simulink model "e03_MtrCtrl_MtrCtrl"  (R2024a)
settings: Solver=FixedStepDiscrete  StartTime=0.0  StopTime=1  FixedStep=mSim.dTime  MaxStep=Define.sModelSampleTime  RelTol=7.1420e-05
undefined symbols (not defined in the file): CnstCnst, CnstMde, CnstNr, E03CCTRL, E03INIT, E03LIM, E03MCMV, sTempGain
libraries: Lib_LPF x2
(part 3 of 3)

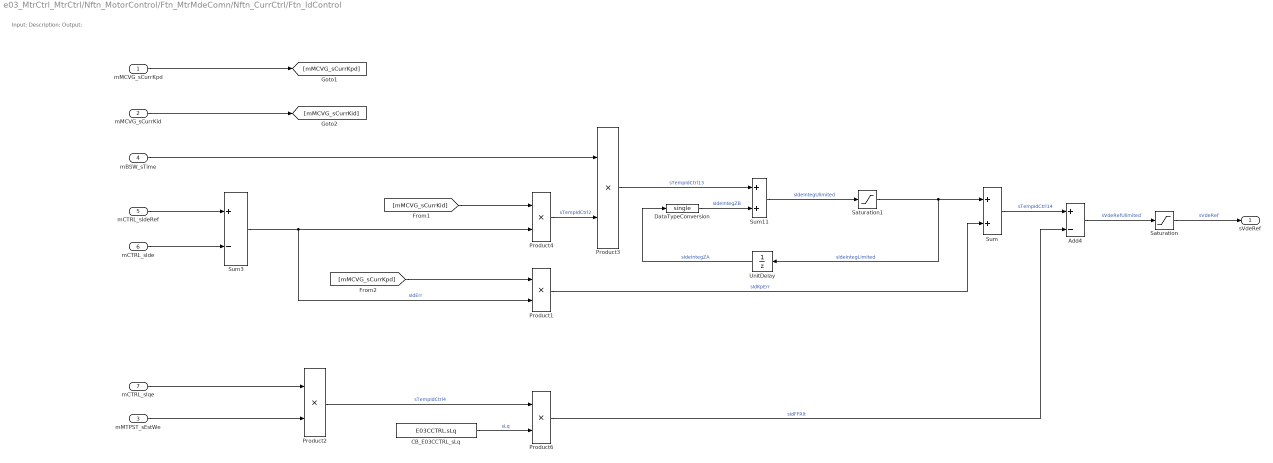
== system e03_MtrCtrl_MtrCtrl/Nftn_MotorControl/Ftn_MtrMdeComn/Nftn_CurrCtrl/Ftn_IdControl ==
  note: Input:
      | Description:
      | Output:
  mMCVG_sCurrKpd : Inport  Description=■ 설명: Current Gain Kp Gain  OutMin=0  OutMax=100
      settings: AttributesFormatString=%<Description>
  mMCVG_sCurrKid : Inport  Description=■ 설명: Current Gain Ki Gain  Port=2  OutMin=0  OutMax=100
      settings: AttributesFormatString=%<Description>
  mMTPST_sEstWe : Inport  Description=■ 설명: 전기 각속도 (We = Wm * Poles)  Port=3  OutMin=0  OutMax=5026.55
      settings: AttributesFormatString=%<Description>
  mBSW_sTime : Inport  Description=■ 설명: 주기, sTime (1/14kH)  Port=4  OutMin=0  OutMax=0.0000714286
      settings: AttributesFormatString=%<Description>
  mCTRL_sIdeRef : Inport  Description=■ 설명: d축 전류 지령  Port=5  OutMin=-49.498  OutMax=49.498
      settings: AttributesFormatString=%<Description>
  mCTRL_sIde : Inport  Description=■ 설명: d축 전류  Port=6  OutMin=-398.3  OutMax=398.3
      settings: AttributesFormatString=%<Description>
  mCTRL_sIqe : Inport  Description=■ 설명: q축 전류  Port=7  OutMin=-398.3  OutMax=398.3
      settings: AttributesFormatString=%<Description>
  Add4 : Sum  Inputs=+-
  CB_E03CCTRL_sLq : Constant  Value=E03CCTRL.sLq
  DataTypeConversion : DataTypeConversion  OutDataTypeStr=single  SaturateOnIntegerOverflow=off  RndMeth=Floor
  Product{1..4,6} (5 alike) : Product
  Saturation : Saturate  UpperLimit=E03LIM.sVrefLim  LowerLimit=E03LIM.sNegVrefLim
      settings: AttributesFormatString=|
      | %<LowerLimit>
      | %<UpperLimit>
  Saturation1 : Saturate  UpperLimit=E03LIM.sVrefLim  LowerLimit=E03LIM.sNegVrefLim
      settings: AttributesFormatString=|
      | %<LowerLimit>
      | %<UpperLimit>
  Sum : Sum
  Sum11 : Sum
  Sum3 : Sum  Inputs=+-
  UnitDelay : UnitDelay  InitialCondition=E03INIT.sIdeCtrlIntegZ  SampleTime=-1  StateName=sIdeIntegZ  HasFrameUpgradeWarning=on
      settings: AttributesFormatString=%<InitialCondition>
  sVdeRef : Outport  Description=■ 설명: d축 전압 지령  OutMin=-1000  OutMax=1000  VectorParamsAs1DForOutWhenUnconnected=off
      settings: AttributesFormatString=%<Description>
  wires:
  Saturation1/1 -> Sum/1, UnitDelay/1  "sIdeIntegLimited"
  Add4/1 -> Saturation/1  "sVdeRefUlimited"
  Product4/1 -> Product3/2  "sTempIdCtrl2"
  Sum3/1 -> Product1/2, Product4/2  "sIdErr"
  Product2/1 -> Product6/1  "sTempIdCtrl4"
  Product1/1 -> Sum/2  "sIdKpErr"
  Product3/1 -> Sum11/1  "sTempIdCtrl13"
  UnitDelay/1 -> DataTypeConversion/1  "sIdeIntegZA"
  mBSW_sTime/1 -> Product3/1
  CB_E03CCTRL_sLq/1 -> Product6/2  "sLq"
  Sum/1 -> Add4/1  "sTempIdCtrl14"
  [mMCVG_sCurrKpd] -> Product1/1
  [mMCVG_sCurrKid] -> Product4/1
  DataTypeConversion/1 -> Sum11/2  "sIdeIntegZB"
  Saturation/1 -> sVdeRef/1  "sVdeRef"
  mMCVG_sCurrKpd/1 -> [mMCVG_sCurrKpd]
  mMCVG_sCurrKid/1 -> [mMCVG_sCurrKid]
  mCTRL_sIdeRef/1 -> Sum3/1
  mCTRL_sIde/1 -> Sum3/2
  mCTRL_sIqe/1 -> Product2/1
  mMTPST_sEstWe/1 -> Product2/2
  Sum11/1 -> Saturation1/1  "sIdeIntegUlimited"
  Product6/1 -> Add4/2  "sIdFFRlt"

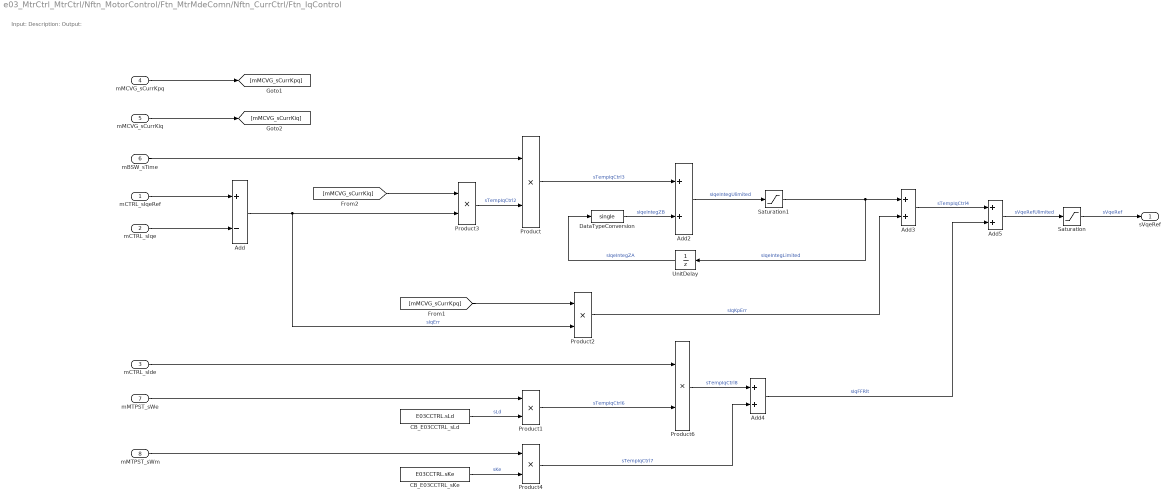
== system e03_MtrCtrl_MtrCtrl/Nftn_MotorControl/Ftn_MtrMdeComn/Nftn_CurrCtrl/Ftn_IqControl ==
  note: Input:
      | Description:
      | Output:
  mCTRL_sIqeRef : Inport  Description=■ 설명: q축 전류 지령  OutMin=-49.498  OutMax=49.498
      settings: AttributesFormatString=%<Description>
  mCTRL_sIqe : Inport  Description=■ 설명: q축 전류  Port=2  OutMin=-398.3  OutMax=398.3
      settings: AttributesFormatString=%<Description>
  mCTRL_sIde : Inport  Description=■ Ide 전류  Port=3  OutMin=-398.3  OutMax=398.3
      settings: AttributesFormatString=%<Description>
  mMCVG_sCurrKpq : Inport  Description=■ 설명: Current Gain Kp Gain  Port=4  OutMin=0  OutMax=100
      settings: AttributesFormatString=%<Description>
  mMCVG_sCurrKiq : Inport  Description=■ 설명: Current Gain Ki Gain  Port=5  OutMin=0  OutMax=100
      settings: AttributesFormatString=%<Description>
  mBSW_sTime : Inport  Description=■ 설명: 주기, sTime (1/14kH)  Port=6  OutMin=0  OutMax=0.0000714286
      settings: AttributesFormatString=%<Description>
  mMTPST_sWe : Inport  Description=■ 설명: 전기 각속도 (We = Wm * Poles)  Port=7  OutMin=0  OutMax=5026.55
      settings: AttributesFormatString=%<Description>
  mMTPST_sWm : Inport  Description=■ 설명: 기계 각속도 (Wm = 12000 * 2pi/60)  Port=8  OutMin=0  OutMax=1256.63706
      settings: AttributesFormatString=%<Description>
  Add : Sum  Inputs=+-
  Add{2..5} (4 alike) : Sum
  CB_E03CCTRL_sKe : Constant  Value=E03CCTRL.sKe
  CB_E03CCTRL_sLd : Constant  Value=E03CCTRL.sLd
  DataTypeConversion : DataTypeConversion  OutDataTypeStr=single  SaturateOnIntegerOverflow=off  RndMeth=Floor
  Product{,1..4,6} (6 alike) : Product
  Saturation : Saturate  UpperLimit=E03LIM.sVrefLim  LowerLimit=E03LIM.sNegVrefLim
      settings: AttributesFormatString=|
      | %<LowerLimit>
      | %<UpperLimit>
  Saturation1 : Saturate  UpperLimit=E03LIM.sVrefLim  LowerLimit=E03LIM.sNegVrefLim
      settings: AttributesFormatString=|
      | %<LowerLimit>
      | %<UpperLimit>
  UnitDelay : UnitDelay  InitialCondition=E03INIT.sIqeCtrlIntegZ  SampleTime=-1  StateName=sIqeIntegZ  HasFrameUpgradeWarning=on
      settings: AttributesFormatString=%<InitialCondition>
  sVqeRef : Outport  Description=■ 설명: q축 전압 지령  OutMin=-1000  OutMax=1000  VectorParamsAs1DForOutWhenUnconnected=off
      settings: AttributesFormatString=%<Description>
  wires:
  Add3/1 -> Add5/1  "sTempIqCtrl4"
  Add/1 -> Product2/2, Product3/2  "sIqErr"
  Add5/1 -> Saturation/1  "sVqeRefUlimited"
  Product2/1 -> Add3/2  "sIqKpErr"
  Add4/1 -> Add5/2  "sIqFFRlt"
  Product6/1 -> Add4/1  "sTempIqCtrl8"
  Saturation1/1 -> UnitDelay/1, Add3/1  "sIqeIntegLimited"
  Product/1 -> Add2/1  "sTempIqCtrl3"
  mBSW_sTime/1 -> Product/1
  Product3/1 -> Product/2  "sTempIqCtrl2"
  [mMCVG_sCurrKiq] -> Product3/1
  Product4/1 -> Add4/2  "sTempIqCtrl7"
  CB_E03CCTRL_sLd/1 -> Product1/2  "sLd"
  CB_E03CCTRL_sKe/1 -> Product4/2  "sKe"
  Product1/1 -> Product6/2  "sTempIqCtrl6"
  [mMCVG_sCurrKpq] -> Product2/1
  UnitDelay/1 -> DataTypeConversion/1  "sIqeIntegZA"
  DataTypeConversion/1 -> Add2/2  "sIqeIntegZB"
  Saturation/1 -> sVqeRef/1  "sVqeRef"
  mMCVG_sCurrKpq/1 -> [mMCVG_sCurrKpq]
  mMCVG_sCurrKiq/1 -> [mMCVG_sCurrKiq]
  mMTPST_sWe/1 -> Product1/1
  mMTPST_sWm/1 -> Product4/1
  mCTRL_sIqeRef/1 -> Add/1
  mCTRL_sIqe/1 -> Add/2
  mCTRL_sIde/1 -> Product6/1
  Add2/1 -> Saturation1/1  "sIqeIntegUlimited"

== system e03_MtrCtrl_MtrCtrl/Nftn_MotorControl/Ftn_MtrMdeComn/Nftn_CurrCtrl/Nftn_GenMuxVdqeRef ==
  note: Input:
      | Description:
      | Output:
  sVdeRef : Inport
  sTheta : Inport  Port=2
  sVqeRef : Inport  Port=3
  Mux : Mux  Inputs=3
  sVdqeRef : Outport
  wires:
  Mux/1 -> sVdqeRef/1  "sVdqeRef"
  sTheta/1 -> Mux/3
  sVqeRef/1 -> Mux/2
  sVdeRef/1 -> Mux/1

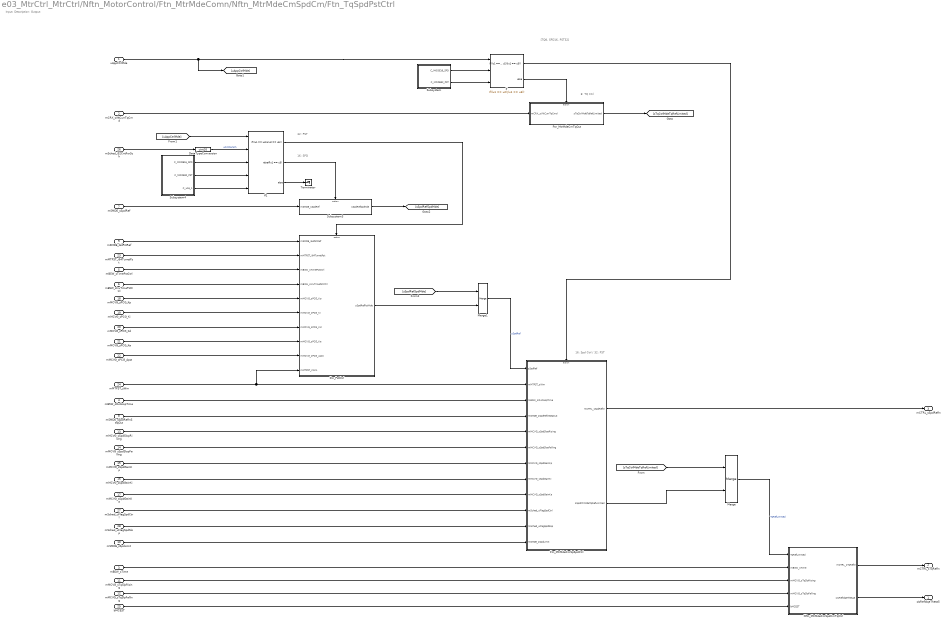
== system e03_MtrCtrl_MtrCtrl/Nftn_MotorControl/Ftn_MtrMdeComn/Nftn_MtrMdeCmSpdCm/Ftn_TqSpdPstCtrl ==
  note: 8: TQ Ctrl
  note: Input:
      | Description:
      | Output:
  note: 16: Spd Ctrl / 32: PST
  note: [TQ8, SPD16, PST32]
  note: 16: SPD
  note: 32: PST
  uAppCtrlMde : Inport  Description=■ 설명: 모터 구동 제어 모드  OutMin=0  OutMax=32
      settings: AttributesFormatString=%<Description>
  mCRX_sVltCurrTqCmd : Inport  Description=■ 설명: uVltCurrTqCmd(Voltage / Current / Torque Reference)  Port=2  OutMin=-398.3  OutMax=398.3
      settings: AttributesFormatString=%<Description>
  mBSW_sTime : Inport  Port=3
  mBSW_sOutloopTime : Inport  Description=■ 설명: sTime * 10  Port=4  OutMin=0  OutMax=0.000714286
      settings: AttributesFormatString=%<Description>
  mBSW_sTimePstCtrl : Inport  Description=■ 설명: sTime * 100  Port=5
      settings: AttributesFormatString=%<Description>
  mBSW_sInvTimePstCtrl : Inport  Description=■ 설명: mBSW_sTimePstCtrl의 역수  Port=6
      settings: AttributesFormatString=%<Description>
  mSMDE_sSpdRef : Inport  Description=■ 설명: Speed Reference  Port=7  OutMin=0  OutMax=11000
      settings: AttributesFormatString=%<Description>
  mSMDE_sSpdRefInSeqOut : Inport  Description=■ 설명: Speed Reference Slop Out  Port=8  OutMin=0  OutMax=11000
      settings: AttributesFormatString=%<Description>
  mSMDE_i64PstRef : Inport  Description='■ 설명: Position Reference  Port=9
      settings: AttributesFormatString=%<Description>
  mSMDE_sSpdLimit : Inport  Description='■ 설명: 속도 제한값  Port=10
      settings: AttributesFormatString=%<Description>
  mMCVG_sTqSlpRising : Inport  Port=11
  mMCVG_sTqSlpFalling : Inport  Port=12
  mMCVG_sSpdSlopRising : Inport  Description=■ 설명: Speed Slop Rising Gain  Port=13  OutMin=0  OutMax=3000
      settings: AttributesFormatString=%<Description>
  mMCVG_sSpdSlopFalling : Inport  Description=■ 설명: Speed Slop Falling Gain  Port=14  OutMin=0  OutMax=3000
      settings: AttributesFormatString=%<Description>
  mMCVG_sSpdGainKp : Inport  Description=■ 설명: Speed Gain Kp Gain  Port=15  OutMin=0  OutMax=10
      settings: AttributesFormatString=%<Description>
  mMCVG_sSpdGainKi : Inport  Description=■ 설명: Speed Gain Ki Gain  Port=16  OutMin=0  OutMax=10
      settings: AttributesFormatString=%<Description>
  mMCVG_sSpdGainKa : Inport  Description=■ 설명: Speed Gain Ka Gain  Port=17  OutMin=0  OutMax=100
      settings: AttributesFormatString=%<Description>
  mMCVG_sPCG_Kp : Inport  Description=■ 설명: 위치 제어 게인 Kp  Port=18
      settings: AttributesFormatString=%<Description>
  mMCVG_sPCG_Ki : Inport  Description=■ 설명: 위치 제어 게인 Ki  Port=19
      settings: AttributesFormatString=%<Description>
  mMCVG_sPCG_Kd : Inport  Description=■ 설명: 위치 제어 게인 Kd  Port=20
      settings: AttributesFormatString=%<Description>
  mMCVG_sPCG_Ka : Inport  Description=■ 설명: 위치 제어 게인 Ka  Port=21
      settings: AttributesFormatString=%<Description>
  mMCVG_sPCG_Apst : Inport  Description=■ 설명: 가속도 게인  Port=22
      settings: AttributesFormatString=%<Description>
  mMTPST_i64TurretPst : Inport  Description=■ 설명: Turret Position  Port=23
      settings: AttributesFormatString=%<Description>
  mMTPST_sWm : Inport  Description=■ 설명: 기계 각속도 (Wm = 2000 * 2pi/60)  Port=24  OutMin=0  OutMax=1256.63706
      settings: AttributesFormatString=%<Description>
  bMCEST : Inport  Port=25
  mSched_i32CntForSch : Inport  Port=26
  mSched_uFlagSpdCtrl : Inport  Description=■ 설명: Speed Control 스케쥴 카운터  Port=27  OutMin=0  OutMax=1
      settings: AttributesFormatString=%<Description>
  mSched_uFlagSpdSlop : Inport  Description=■ 설명: 속도 지령 Slop 스케쥴 카운터  Port=28  OutMin=0  OutMax=1
      settings: AttributesFormatString=%<Description>
  DataTypeConversion : DataTypeConversion  OutDataTypeStr=uint16  SaturateOnIntegerOverflow=off  RndMeth=Floor
  Ftn_MtrMdeCmSpSpdCtrl : Subsystem
      settings: RTWSystemCode=Nonreusable function  RTWFcnNameOpts=Use subsystem name
  Ftn_MtrMdeCmTqOut : Subsystem
  Ftn_PstCtrl : Subsystem
      settings: RTWSystemCode=Nonreusable function  RTWFcnNameOpts=Use subsystem name
  If : If  NumInputs=3  IfExpression=(u1 == u2)|(u1 == u3)
  If1 : If  NumInputs=5  IfExpression=(u1 == u4)&(u2 == u5)  ElseIfExpressions=u1 == u3
  Merge : Merge
  Merge1 : Merge
  Nftn_MtrMdeCmSpdCmTqCtrl : Subsystem
  Subsystem : Subsystem
  Subsystem3 : Subsystem
  Subsystem4 : Subsystem
  Terminator : Terminator
  sIsRefIdqeTheta5 : Outport  Description=|  OutMin=-398.3  OutMax=398.3
      | ■ 설명: 제어 모드 전류 출력 Mux 신호
      | -.[0] : 전압/전류/토크 지령
      | -.[1] : d축 전류
      | -.[2] : q축 전류
      | -.[3] : 추정 위치
      settings: AttributesFormatString=%<Description>
  mCTRL_sTqRefIn : Outport  Description=■ 설명: Tq Slop Reference  Port=2  OutMin=-398.3  OutMax=398.3
      settings: AttributesFormatString=%<Description>
  mCTRL_sSpdRefIn : Outport  Description=■ 설명: Speed Reference  Port=3  OutMin=0  OutMax=11000
      settings: AttributesFormatString=%<Description>
  wires:
  [sTqCtrlMdeTqRefLimited] -> Merge/1
  If/1 -> Ftn_MtrMdeCmSpSpdCtrl/Action
  uAppCtrlMde/1 -> [uAppCtrlMde], If/1
  If/2 -> Ftn_MtrMdeCmTqOut/Action
  Ftn_MtrMdeCmSpSpdCtrl/1(mCTRL_sSpdRefIn) -> mCTRL_sSpdRefIn/1
  Nftn_MtrMdeCmSpdCmTqCtrl/2(sIsRefIdqeTheta5) -> sIsRefIdqeTheta5/1
  Ftn_MtrMdeCmTqOut/1(sTqCtrlMdeTqRefLimited) -> [sTqCtrlMdeTqRefLimited]
  mBSW_sOutloopTime/1 -> Ftn_MtrMdeCmSpSpdCtrl/3(mBSW_sOutloopTime)
  mSMDE_sSpdRef/1 -> Subsystem3/1(mSMDE_sSpdRef)
  mSMDE_sSpdRefInSeqOut/1 -> Ftn_MtrMdeCmSpSpdCtrl/4(mSMDE_sSpdRefInSeqOut)
  mCRX_sVltCurrTqCmd/1 -> Ftn_MtrMdeCmTqOut/1(mCRX_sVltCurrTqCmd)
  mMCVG_sSpdSlopRising/1 -> Ftn_MtrMdeCmSpSpdCtrl/5(mMCVG_sSpdSlopRising)
  mMCVG_sSpdSlopFalling/1 -> Ftn_MtrMdeCmSpSpdCtrl/6(mMCVG_sSpdSlopFalling)
  mMCVG_sSpdGainKp/1 -> Ftn_MtrMdeCmSpSpdCtrl/7(mMCVG_sSpdGainKp)
  mMCVG_sSpdGainKi/1 -> Ftn_MtrMdeCmSpSpdCtrl/8(mMCVG_sSpdGainKi)
  mMCVG_sSpdGainKa/1 -> Ftn_MtrMdeCmSpSpdCtrl/9(mMCVG_sSpdGainKa)
  mMTPST_sWm/1 -> Ftn_PstCtrl/10(mMTPST_sWm), Ftn_MtrMdeCmSpSpdCtrl/2(mMTPST_sWm)
  mSched_uFlagSpdCtrl/1 -> Ftn_MtrMdeCmSpSpdCtrl/10(mSched_uFlagSpdCtrl)
  mSched_uFlagSpdSlop/1 -> Ftn_MtrMdeCmSpSpdCtrl/11(mSched_uFlagSpdSlop)
  bMCEST/1 -> Nftn_MtrMdeCmSpdCmTqCtrl/5(bMCEST)
  Ftn_MtrMdeCmSpSpdCtrl/2(sSpdCtrlMdeTqRefLimited) -> Merge/2
  Nftn_MtrMdeCmSpdCmTqCtrl/1(mCTRL_sTqRefIn) -> mCTRL_sTqRefIn/1
  mMCVG_sTqSlpFalling/1 -> Nftn_MtrMdeCmSpdCmTqCtrl/4(mMCVG_sTqSlpFalling)
  mMCVG_sTqSlpRising/1 -> Nftn_MtrMdeCmSpdCmTqCtrl/3(mMCVG_sTqSlpRising)
  mBSW_sTime/1 -> Nftn_MtrMdeCmSpdCmTqCtrl/2(mBSW_sTime)
  Merge/1 -> Nftn_MtrMdeCmSpdCmTqCtrl/1(TqRefLimited)  "TqRefLimited"
  Subsystem/1(C_MODE16_SPD) -> If/2
  Subsystem/2(C_MODE32_PST) -> If/3
  [uAppCtrlMde] -> If1/1
  Subsystem4/1(C_MODE16_SPD) -> If1/3
  Subsystem4/2(C_MODE32_PST) -> If1/4
  Subsystem3/1(sSpdRefSpdMde) -> [sSpdRefSpdMde]
  Ftn_PstCtrl/1(sSpdRefPstMde) -> Merge1/2
  Merge1/1 -> Ftn_MtrMdeCmSpSpdCtrl/1(sSpdRef)  "sSpdRef"
  [sSpdRefSpdMde] -> Merge1/1
  mMCVG_sPCG_Kp/1 -> Ftn_PstCtrl/5(mMCVG_sPCG_Kp)
  mMCVG_sPCG_Ki/1 -> Ftn_PstCtrl/6(mMCVG_sPCG_Ki)
  mMCVG_sPCG_Kd/1 -> Ftn_PstCtrl/7(mMCVG_sPCG_Kd)
  mMCVG_sPCG_Ka/1 -> Ftn_PstCtrl/8(mMCVG_sPCG_Ka)
  mMCVG_sPCG_Apst/1 -> Ftn_PstCtrl/9(mMCVG_sPCG_Apst)
  mBSW_sTimePstCtrl/1 -> Ftn_PstCtrl/3(mBSW_sTimePstCtrl)
  If1/2 -> Subsystem3/Action
  If1/1 -> Ftn_PstCtrl/Action
  mSched_i32CntForSch/1 -> DataTypeConversion/1
  If1/3 -> Terminator/1
  Subsystem4/3(C_u16_1) -> If1/5
  mSMDE_i64PstRef/1 -> Ftn_PstCtrl/1(mSMDE_i64PstRef)
  mMTPST_i64TurretPst/1 -> Ftn_PstCtrl/2(mMTPST_i64TurretPst)
  DataTypeConversion/1 -> If1/2  "uCntForSch"
  mBSW_sInvTimePstCtrl/1 -> Ftn_PstCtrl/4(mBSW_sInvTimePstCtrl)
  mSMDE_sSpdLimit/1 -> Ftn_MtrMdeCmSpSpdCtrl/12(mSMDE_sSpdLimit)

== system e03_MtrCtrl_MtrCtrl/Nftn_MotorControl/Ftn_MtrMdeComn/Ftn_CurrRefSelection/Nftn_SftCurrMde/Nftn_CalIsBeta2IdqRef ==
  note: Input:
      | Description:
      | Output:
  mCTRL_sIsRefIn : Inport
  mCRX_sFreqBetaCmd : Inport  Port=2
  uAppCtrlMde : Inport  Port=3
  BusCreator : BusCreator  Inputs=2
  CB_C_90 : Constant  Value=CnstCnst.C_90
  CB_C_MODE32_IF : Constant  Value=CnstMde.C_MODE256_IF
  CB_C_MODE64_VALIGN : Constant  Value=CnstMde.C_MODE64_VALIGN
  CB_C_PI2_INV_360 : Constant  Value=CnstCnst.C_PI2_INV_360
  CB_sBetaRiseStep : Constant  Value=E03MCMV.sBetaRiseStep
  CB_sMaxFreq : Constant  Value=E03MCMV.sMaxFreq
  CB_sZero : Constant  Value=0  OutDataTypeStr=single
  Chart_CalIsBeta2IdqRef : Stateflow chart  TreatAsAtomicUnit=on
  Terminator : Terminator
  sIdqeRef : Outport
  wires:
  Chart_CalIsBeta2IdqRef/1(sIdeRefCurrMde) -> BusCreator/1
  Chart_CalIsBeta2IdqRef/2(sIqeRefCurrMde) -> BusCreator/2
  mCTRL_sIsRefIn/1 -> Chart_CalIsBeta2IdqRef/1(mCTRL_sIsRefIn)
  BusCreator/1 -> sIdqeRef/1  "sIdqeRef"
  uAppCtrlMde/1 -> Chart_CalIsBeta2IdqRef/3(uAppCtrlMde)
  CB_C_90/1 -> Chart_CalIsBeta2IdqRef/4(C_90)  "C_90"
  CB_C_MODE64_VALIGN/1 -> Chart_CalIsBeta2IdqRef/5(C_MODE64_VALIGN)  "C_MODE64_VALIGN"
  CB_C_MODE32_IF/1 -> Chart_CalIsBeta2IdqRef/6(C_MODE256_IF)  "C_MODE256_IF"
  CB_C_PI2_INV_360/1 -> Chart_CalIsBeta2IdqRef/7(C_PI2_INV_360)  "C_PI2_INV_360"
  CB_sBetaRiseStep/1 -> Chart_CalIsBeta2IdqRef/8(sBetaRiseStep)  "sBetaRiseStep"
  CB_sZero/1 -> Chart_CalIsBeta2IdqRef/10(sZero)  "sZero"
  Chart_CalIsBeta2IdqRef/3(sIFreqBetaCmd) -> Terminator/1
  mCRX_sFreqBetaCmd/1 -> Chart_CalIsBeta2IdqRef/2(mCRX_sFreqBetaCmd)
  CB_sMaxFreq/1 -> Chart_CalIsBeta2IdqRef/9(sMaxFreq)  "sMaxFreq"

== system e03_MtrCtrl_MtrCtrl/Nftn_MotorControl/Ftn_MtrMdeComn/Ftn_CurrRefSelection/Nftn_SftCurrMde/Nftn_GensAppIeRefLim ==
  note: Input:
      | Description:
      | Output:
  mCTRL_sIsRef : Inport
  CB_E03LIM_sCurrLim : Constant  Value=E03LIM.sCurrLim
  Chart_GensAppIeRefLim : Stateflow chart  TreatAsAtomicUnit=on
  sIsRefLimed : Outport
  wires:
  Chart_GensAppIeRefLim/1(sIsRefLimed) -> sIsRefLimed/1
  CB_E03LIM_sCurrLim/1 -> Chart_GensAppIeRefLim/2(sCurrLim)  "sCurrLim"
  mCTRL_sIsRef/1 -> Chart_GensAppIeRefLim/1(mCTRL_sIsRef)

== system e03_MtrCtrl_MtrCtrl/Nftn_MotorControl/Ftn_MtrMdeComn/Ftn_CurrRefSelection/Nftn_SftCurrMde/Nftn_SftMdeCurrBypass ==
  note: Input:
      | Description:
      | Output:
  sIsRefLimed : Inport
  ActionPort : ActionPort  ActionPortLabel=default:
  SignalConversion : SignalConversion  OverrideOpt=off
  sIsRefIn1 : Outport  VectorParamsAs1DForOutWhenUnconnected=off
  wires:
  SignalConversion/1 -> sIsRefIn1/1  "sIsRefIn1"
  sIsRefLimed/1 -> SignalConversion/1

== system e03_MtrCtrl_MtrCtrl/Nftn_MotorControl/Ftn_MtrMdeComn/Ftn_CurrRefSelection/Nftn_SftCurrMde/Nftn_SftMdeCurrStart ==
  note: Input:
      | Description:
      | Output:
  sIsRefLimed : Inport
  mBSW_sTime : Inport  Port=2
  mMCVG_sCurrSlopRising : Inport  Port=3
  mMCVG_sCurrSlopFalling : Inport  Port=4
  ActionPort : ActionPort  ActionPortLabel=case [ 2 ]:
  Product : Product
  Product1 : Product
  RelationalOperator1 : RelationalOperator  Operator=<  InputSameDT=off
  RelationalOperator2 : RelationalOperator  Operator=>  InputSameDT=off
  Sum : Sum
  Sum1 : Sum  Inputs=+-
  Switch1 : Switch  Criteria=u2 ~= 0  SaturateOnIntegerOverflow=off  InputSameDT=off
  Switch2 : Switch  Criteria=u2 ~= 0  SaturateOnIntegerOverflow=off  InputSameDT=off
  UnitDelay_sIsRefIn : UnitDelay  InitialCondition=E03INIT.sIsRefInZ  SampleTime=-1  StateName=sIsRefIn2  HasFrameUpgradeWarning=on
      settings: AttributesFormatString=%<InitialCondition>
  sIsRefIn2 : Outport  VectorParamsAs1DForOutWhenUnconnected=off
  wires:
  UnitDelay_sIsRefIn/1 -> [sIsRefIn2Z]  "sIsRefIn2Z"
  Switch2/1 -> UnitDelay_sIsRefIn/1, sIsRefIn2/1  "sIsRefIn2"
  sIsRefLimed/1 -> RelationalOperator1/1, Switch1/1
  Switch1/1 -> Switch2/1, RelationalOperator2/1  "sBudMax2"
  [sIsRefIn2Z] -> Sum1/1, Sum/2
  Sum1/1 -> RelationalOperator2/2, Switch2/3  "sBaudMin"
  RelationalOperator1/1 -> Switch1/2  "sTempSftCurr1"
  RelationalOperator2/1 -> Switch2/2  "sTempSftCurr2"
  Product1/1 -> Sum1/2  "sStepFalling"
  Product/1 -> Sum/1  "sStepRising"
  Sum/1 -> RelationalOperator1/2, Switch1/3  "sBaudMax1"
  mMCVG_sCurrSlopFalling/1 -> Product1/2
  mMCVG_sCurrSlopRising/1 -> Product/2
  [mBSW_sTime] -> Product1/1
  mBSW_sTime/1 -> [mBSW_sTime], Product/1

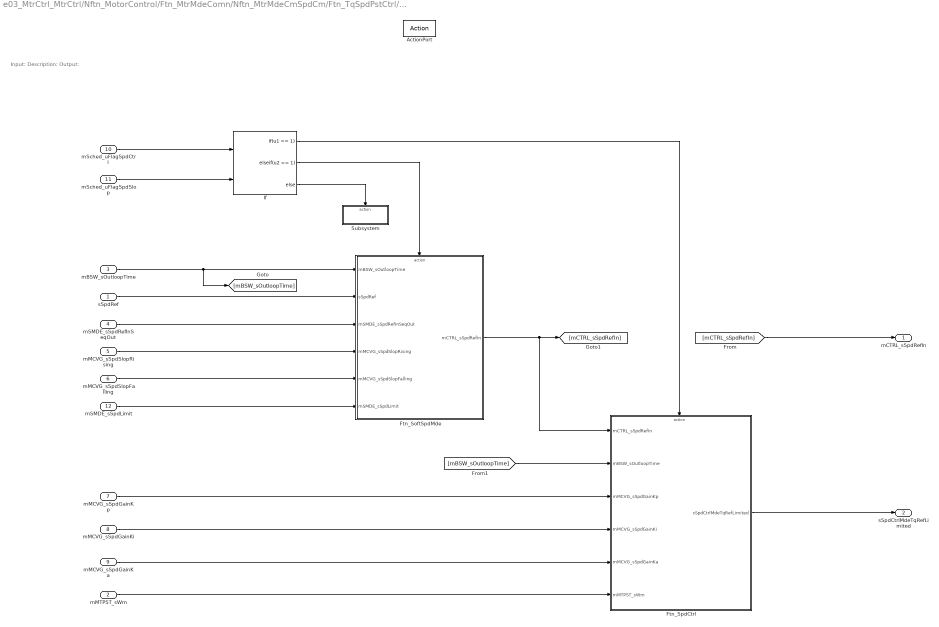
== system e03_MtrCtrl_MtrCtrl/Nftn_MotorControl/Ftn_MtrMdeComn/Nftn_MtrMdeCmSpdCm/Ftn_TqSpdPstCtrl/Ftn_MtrMdeCmSpSpdCtrl ==
  note: Input:
      | Description:
      | Output:
  sSpdRef : Inport  Description=■ 설명: Speed Reference  OutMin=0  OutMax=11000
      settings: AttributesFormatString=%<Description>
  mMTPST_sWm : Inport  Description=■ 설명: 기계 각속도 (Wm = 12000 * 2pi/60)  Port=2  OutMin=0  OutMax=1256.63706
      settings: AttributesFormatString=%<Description>
  mBSW_sOutloopTime : Inport  Description=■ 설명: sTime * 10  Port=3  OutMin=0  OutMax=0.000714286
      settings: AttributesFormatString=%<Description>
  mSMDE_sSpdRefInSeqOut : Inport  Description=■ 설명: Speed Reference Slop Out  Port=4  OutMin=0  OutMax=11000
      settings: AttributesFormatString=%<Description>
  mMCVG_sSpdSlopRising : Inport  Description=■ 설명: Speed Slop Rising Gain  Port=5  OutMin=0  OutMax=3000
      settings: AttributesFormatString=%<Description>
  mMCVG_sSpdSlopFalling : Inport  Description=■ 설명: Speed Slop Falling Gain  Port=6  OutMin=0  OutMax=3000
      settings: AttributesFormatString=%<Description>
  mMCVG_sSpdGainKp : Inport  Description=■ 설명: Speed Gain Kp Gain  Port=7  OutMin=0  OutMax=10
      settings: AttributesFormatString=%<Description>
  mMCVG_sSpdGainKi : Inport  Description=■ 설명: Speed Gain Ki Gain  Port=8  OutMin=0  OutMax=10
      settings: AttributesFormatString=%<Description>
  mMCVG_sSpdGainKa : Inport  Description=■ 설명: Speed Gain Ka Gain  Port=9  OutMin=0  OutMax=100
      settings: AttributesFormatString=%<Description>
  mSched_uFlagSpdCtrl : Inport  Description=■ 설명: Speed Control 스케쥴 카운터  Port=10  OutMin=0  OutMax=1
      settings: AttributesFormatString=%<Description>
  mSched_uFlagSpdSlop : Inport  Description=■ 설명: 속도 지령 Slop 스케쥴 카운터  Port=11  OutMin=0  OutMax=1
      settings: AttributesFormatString=%<Description>
  mSMDE_sSpdLimit : Inport  Description='■ 설명: 속도 제한값  Port=12
      settings: AttributesFormatString=%<Description>
  ActionPort : ActionPort  ActionPortLabel=if((u1 == u2)|(u1 == u3))
  Ftn_SoftSpdMde : Subsystem
      settings: RTWSystemCode=Nonreusable function  RTWFcnNameOpts=Use subsystem name
  Ftn_SpdCtrl : Subsystem  Description="/*  d-Axis Current Control  */"  TreatAsAtomicUnit=on
      settings: RTWSystemCode=Nonreusable function  RTWFcnNameOpts=Use subsystem name
  If : If  NumInputs=2  IfExpression=u1 == 1  ElseIfExpressions=u2 == 1
  Subsystem : Subsystem
  mCTRL_sSpdRefIn : Outport  Description=■ 설명: Speed Reference  OutMin=0  OutMax=11000
      settings: AttributesFormatString=%<Description>
  sSpdCtrlMdeTqRefLimited : Outport  Description=■ 설명: Tq Slop Reference  Port=2  OutMin=-12577.8  OutMax=12577.8  VectorParamsAs1DForOutWhenUnconnected=off
      settings: AttributesFormatString=%<Description>
  wires:
  Ftn_SoftSpdMde/1(mCTRL_sSpdRefIn) -> Ftn_SpdCtrl/1(mCTRL_sSpdRefIn), [mCTRL_sSpdRefIn]
  Ftn_SpdCtrl/1(sSpdCtrlMdeTqRefLimited) -> sSpdCtrlMdeTqRefLimited/1
  [mCTRL_sSpdRefIn] -> mCTRL_sSpdRefIn/1
  If/3 -> Subsystem/Action
  If/2 -> Ftn_SoftSpdMde/Action
  mSched_uFlagSpdCtrl/1 -> If/1
  mSched_uFlagSpdSlop/1 -> If/2
  If/1 -> Ftn_SpdCtrl/Action
  mBSW_sOutloopTime/1 -> Ftn_SoftSpdMde/1(mBSW_sOutloopTime), [mBSW_sOutloopTime]
  [mBSW_sOutloopTime] -> Ftn_SpdCtrl/2(mBSW_sOutloopTime)
  sSpdRef/1 -> Ftn_SoftSpdMde/2(sSpdRef)
  mSMDE_sSpdRefInSeqOut/1 -> Ftn_SoftSpdMde/3(mSMDE_sSpdRefInSeqOut)
  mMCVG_sSpdSlopRising/1 -> Ftn_SoftSpdMde/4(mMCVG_sSpdSlopRising)
  mMCVG_sSpdSlopFalling/1 -> Ftn_SoftSpdMde/5(mMCVG_sSpdSlopFalling)
  mMCVG_sSpdGainKp/1 -> Ftn_SpdCtrl/3(mMCVG_sSpdGainKp)
  mMCVG_sSpdGainKi/1 -> Ftn_SpdCtrl/4(mMCVG_sSpdGainKi)
  mMCVG_sSpdGainKa/1 -> Ftn_SpdCtrl/5(mMCVG_sSpdGainKa)
  mMTPST_sWm/1 -> Ftn_SpdCtrl/6(mMTPST_sWm)
  mSMDE_sSpdLimit/1 -> Ftn_SoftSpdMde/6(mSMDE_sSpdLimit)

== system e03_MtrCtrl_MtrCtrl/Nftn_MotorControl/Ftn_MtrMdeComn/Nftn_MtrMdeCmSpdCm/Ftn_TqSpdPstCtrl/Ftn_MtrMdeCmTqOut ==
  mCRX_sVltCurrTqCmd : Inport
  ActionPort : ActionPort  ActionPortLabel=else
  Saturation1 : Saturate  UpperLimit=E03LIM.sMaxTqSet  LowerLimit=E03LIM.sNegMaxTqSet
      settings: AttributesFormatString=|
      | %<LowerLimit>
      | %<UpperLimit>
  sTqCtrlMdeTqRefLimited : Outport
  wires:
  Saturation1/1 -> sTqCtrlMdeTqRefLimited/1  "sTqCtrlMdeTqRefLimited"
  mCRX_sVltCurrTqCmd/1 -> Saturation1/1

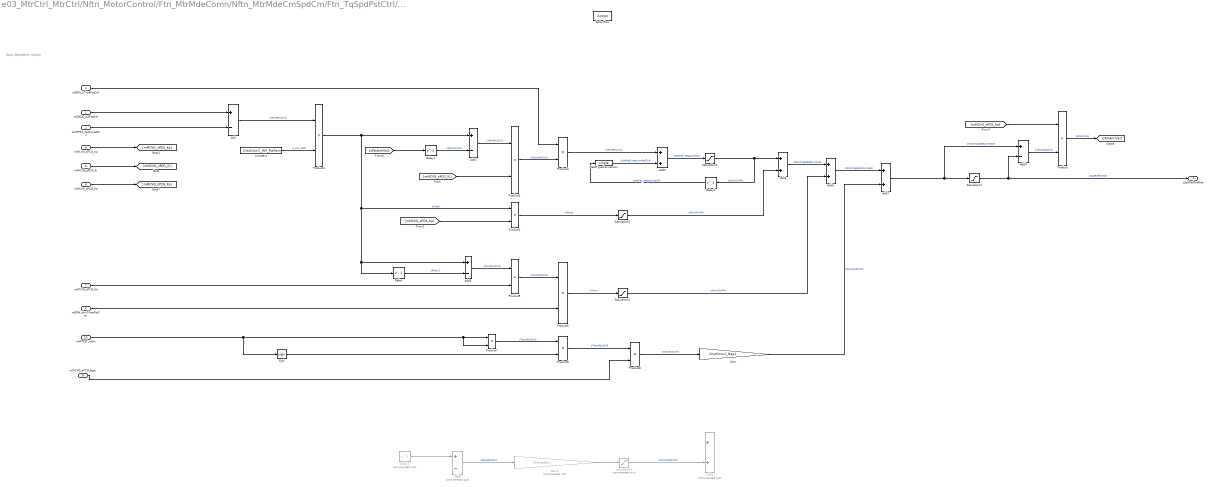
== system e03_MtrCtrl_MtrCtrl/Nftn_MotorControl/Ftn_MtrMdeComn/Nftn_MtrMdeCmSpdCm/Ftn_TqSpdPstCtrl/Ftn_PstCtrl ==
  note: Input:
      | Description:
      | Output:
  mSMDE_i64PstRef : Inport  Description=■ 설명: Speed Reference  OutMin=0  OutMax=11000
      settings: AttributesFormatString=%<Description>
  mMTPST_i64TurretPst : Inport  Description=■ 설명: 기계 각속도 (Wm = 12000 * 2pi/60)  Port=2  OutMin=0  OutMax=1256.63706
      settings: AttributesFormatString=%<Description>
  mBSW_sTimePstCtrl : Inport  Description=■ 설명: sTime * 10  Port=3  OutMin=0  OutMax=0.000714286
      settings: AttributesFormatString=%<Description>
  mBSW_sInvTimePstCtrl : Inport  Port=4
  mMCVG_sPCG_Kp : Inport  Description=■ 설명: Speed Gain Kp Gain  Port=5  OutMin=0  OutMax=10
      settings: AttributesFormatString=%<Description>
  mMCVG_sPCG_Ki : Inport  Description=■ 설명: Speed Gain Ki Gain  Port=6  OutMin=0  OutMax=10
      settings: AttributesFormatString=%<Description>
  mMCVG_sPCG_Kd : Inport  Port=7
  mMCVG_sPCG_Ka : Inport  Description=■ 설명: Speed Gain Ka Gain  Port=8  OutMin=0  OutMax=100
      settings: AttributesFormatString=%<Description>
  mMCVG_sPCG_Apst : Inport  Port=9
  mMTPST_sWm : Inport  Description=■ 설명: 기계 각속도 (Wm = 2000 * 2pi/60)  Port=10
      settings: AttributesFormatString=%<Description>
  ActionPort : ActionPort  ActionPortLabel=if((u1 == u4)&(u2 == u5))
  Add{,1,4..5} (4 alike) : Sum  Inputs=+-
  Add{2..3,6..7} (4 alike) : Sum
  Add8 : Sum  Commented=on  Inputs=+-
  Add9 : Sum  Commented=on
  Constant : Constant  Value=CnstCnst.C_INV_PstGain
  DataTypeConversion : DataTypeConversion  OutDataTypeStr=single  SaturateOnIntegerOverflow=off  RndMeth=Floor
  Delay : Delay  DelayLength=1
  Delay1 : Delay  DelayLength=1
  Delay2 : Delay  DelayLength=1
  Delay3 : Delay  Commented=on  DelayLength=1
  Gain : Gain  Gain=CnstCnst.C_Neg1
  Gain1 : Gain  Commented=on  Gain=sTempGain  OutDataTypeStr=single
  Product{,1..9} (10 alike) : Product
  Saturation1 : Saturate  UpperLimit=E03LIM.sMaxSpdSet  LowerLimit=E03LIM.sNegMaxSpdSet
      settings: AttributesFormatString=|
      | %<LowerLimit>
      | %<UpperLimit>
  Saturation2 : Saturate  UpperLimit=E03LIM.sMaxSpdSet*0.05  LowerLimit=E03LIM.sNegMaxSpdSet*0.05
      settings: AttributesFormatString=|
      | %<LowerLimit>
      | %<UpperLimit>
  Saturation3 : Saturate  UpperLimit=E03LIM.sMaxSpdSet*1.5  LowerLimit=E03LIM.sNegMaxSpdSet*1.5
      settings: AttributesFormatString=|
      | %<LowerLimit>
      | %<UpperLimit>
  Saturation4 : Saturate  Commented=on  UpperLimit=E03LIM.sMaxSpdSet  LowerLimit=E03LIM.sNegMaxSpdSet
      settings: AttributesFormatString=|
      | %<LowerLimit>
      | %<UpperLimit>
  Saturation5 : Saturate  UpperLimit=E03LIM.sMaxSpdSet*1.5  LowerLimit=E03LIM.sNegMaxSpdSet*1.5
      settings: AttributesFormatString=|
      | %<LowerLimit>
      | %<UpperLimit>
  Sign : Signum
  sSpdRefPstMde : Outport  Description=■ 설명: 속도 제어기 PI제어 출력값  OutMin=-12577.8  OutMax=12577.8  VectorParamsAs1DForOutWhenUnconnected=off
      settings: AttributesFormatString=%<Description>
  wires:
  [mMCVG_sPCG_Ki] -> Product2/2
  DataTypeConversion/1 -> Add2/2  "sSpdRef_IntegLimitedZAB"
  Delay1/1 -> Add1/2  "sPstAntiValZ"
  mMCVG_sPCG_Ka/1 -> [mMCVG_sPCG_Ka]
  [mMCVG_sPCG_Ka] -> Product/1
  mBSW_sTimePstCtrl/1 -> Product3/1
  Product2/1 -> Product3/2  "sTempPstCtrl3"
  Add4/1 -> Product/2  "sTempSpdCtrl6"
  mMTPST_i64TurretPst/1 -> Add/2
  Add1/1 -> Product2/1  "sTempPstCtrl2"
  Product1/1 -> Saturation5/1  "sTemp1"
  [sPstAntiVal] -> Delay1/1
  mMCVG_sPCG_Ki/1 -> [mMCVG_sPCG_Ki]
  Product3/1 -> Add2/1  "sTempPstCtrl4"
  Product4/1 -> Delay/1, Add5/1, Product1/1, Add1/1  "sPsterr"
  Saturation2/1 -> Delay2/1, Add3/1  "sPstKiCtrlRlt"
  Add2/1 -> Saturation2/1  "sSpdRef_IntegUlimited"
  mMCVG_sPCG_Kp/1 -> [mMCVG_sPCG_Kp]
  Saturation1/1 -> sSpdRefPstMde/1, Add4/2  "sSpdRefPstMde"
  Product/1 -> [sPstAntiVal]  "sPstAntiVal"
  [mMCVG_sPCG_Kp] -> Product1/2
  mSMDE_i64PstRef/1 -> Add/1
  Delay2/1 -> DataTypeConversion/1  "sSpdRef_IntegLimitedZA"
  Constant/1 -> Product4/2  "C_INV_1000"
  Delay/1 -> Add5/2  "sPsterrZ"
  Add5/1 -> Product5/1  "sTempPstCtrl6"
  mMCVG_sPCG_Kd/1 -> Product5/2
  Product5/1 -> Product6/1  "sTempPstCtrl5"
  mBSW_sInvTimePstCtrl/1 -> Product6/2
  Saturation3/1 -> Add6/2  "sPstKdCtrlRlt"
  Add3/1 -> Add6/1  "sPstCtrlSpdRefUlimited1"
  Add6/1 -> Add7/1  "sPstCtrlSpdRefUlimited2"
  mMTPST_sWm/1 -> Sign/1, Product7/2, Product7/1
  Product7/1 -> Product9/1  "sTempPstCtrl5"
  mMCVG_sPCG_Apst/1 -> Product8/2
  Gain/1 -> Add7/2  "sPstApstCtrlRlt"
  Add/1 -> Product4/1  "sTempPstCtrl0"
  Product8/1 -> Gain/1  "sTempPstCtrl6"
  Delay3/1 -> Add8/1
  Add8/1 -> Gain1/1  "sTempPstCtrl7"
  Add7/1 -> Saturation1/1, Add4/1  "sPstCtrlSpdRefUlimited3"
  Saturation4/1 -> Add9/2  "sPstWndtCtrlRlt"
  Gain1/1 -> Saturation4/1
  Product6/1 -> Saturation3/1  "sTemp"
  Saturation5/1 -> Add3/2  "sPstKpCtrlRlt"
  Sign/1 -> Product9/2
  Product9/1 -> Product8/1  "sTempPstCtrl6"

== system e03_MtrCtrl_MtrCtrl/Nftn_MotorControl/Ftn_MtrMdeComn/Nftn_MtrMdeCmSpdCm/Ftn_TqSpdPstCtrl/Nftn_MtrMdeCmSpdCmTqCtrl ==
  note: Input:
      | Description:
      | Output:
  TqRefLimited : Inport
  mBSW_sTime : Inport  Port=2
  mMCVG_sTqSlpRising : Inport  Port=3
  mMCVG_sTqSlpFalling : Inport  Port=4
  bMCEST : Inport  Port=5
  Nftn_SftMdeTqRef : Subsystem
      settings: RTWFcnNameOpts=Use subsystem name
  Nftn_TqLimit : Subsystem
  mCTRL_sTqRefIn : Outport
  sIsRefIdqeTheta5 : Outport  Description=■ 설명: uVltCurrTqCmd(Voltage / Current / Torque Reference)  Port=2  OutMin=-398.3  OutMax=398.3
      settings: AttributesFormatString=%<Description>
  wires:
  mMCVG_sTqSlpFalling/1 -> Nftn_SftMdeTqRef/4(mMCVG_sTqSlpFalling)
  mMCVG_sTqSlpRising/1 -> Nftn_SftMdeTqRef/3(mMCVG_sTqSlpRising)
  TqRefLimited/1 -> Nftn_SftMdeTqRef/1(TqRefLimited)
  mBSW_sTime/1 -> Nftn_SftMdeTqRef/2(mBSW_sTime)
  Nftn_SftMdeTqRef/1(mCTRL_sTqRefIn) -> mCTRL_sTqRefIn/1, Nftn_TqLimit/1(mCTRL_sTqRefIn)
  bMCEST/1 -> Nftn_TqLimit/2(bMCEST)
  Nftn_TqLimit/1(sIsRefIdqeTheta5) -> sIsRefIdqeTheta5/1

== system e03_MtrCtrl_MtrCtrl/Nftn_MotorControl/Ftn_MtrMdeComn/Nftn_MtrMdeCmSpdCm/Ftn_TqSpdPstCtrl/Subsystem ==
  note: Input:
      | Description:
      | Output:
  CB_C_MODE16_SPD : Constant  Value=CnstMde.C_MODE16_SPD
  CB_C_MODE32_PST : Constant  Value=CnstMde.C_MODE32_PST
  C_MODE16_SPD : Outport
  C_MODE32_PST : Outport  Port=2
  wires:
  CB_C_MODE16_SPD/1 -> C_MODE16_SPD/1  "C_MODE16_SPD"
  CB_C_MODE32_PST/1 -> C_MODE32_PST/1  "C_MODE32_PST"

== system e03_MtrCtrl_MtrCtrl/Nftn_MotorControl/Ftn_MtrMdeComn/Nftn_MtrMdeCmSpdCm/Ftn_TqSpdPstCtrl/Subsystem3 ==
  mSMDE_sSpdRef : Inport
  ActionPort : ActionPort  ActionPortLabel=elseif(u1 == u3)
  SignalConversion : SignalConversion  OverrideOpt=off
  sSpdRefSpdMde : Outport
  wires:
  mSMDE_sSpdRef/1 -> SignalConversion/1
  SignalConversion/1 -> sSpdRefSpdMde/1  "sSpdRefSpdMde"

== system e03_MtrCtrl_MtrCtrl/Nftn_MotorControl/Ftn_MtrMdeComn/Nftn_MtrMdeCmSpdCm/Ftn_TqSpdPstCtrl/Subsystem4 ==
  note: Input:
      | Description:
      | Output:
  CB_C_MODE16_SPD : Constant  Value=CnstMde.C_MODE16_SPD
  CB_C_MODE32_PST : Constant  Value=CnstMde.C_MODE32_PST
  CB_C_u16_1 : Constant  Value=CnstNr.C_u16_1
  C_MODE16_SPD : Outport
  C_MODE32_PST : Outport  Port=2
  C_u16_1 : Outport  Port=3
  wires:
  CB_C_MODE32_PST/1 -> C_MODE32_PST/1  "C_MODE32_PST"
  CB_C_MODE16_SPD/1 -> C_MODE16_SPD/1  "C_MODE16_SPD"
  CB_C_u16_1/1 -> C_u16_1/1  "C_u16_1"

== system e03_MtrCtrl_MtrCtrl/Nftn_MotorControl/Ftn_MtrMdeComn/Nftn_MtrMdeCmSpdCm/Ftn_TqSpdPstCtrl/Ftn_MtrMdeCmSpSpdCtrl/Ftn_SoftSpdMde ==
  note: Input:
      | Description:
      | Output:
  mBSW_sOutloopTime : Inport  Description=■ 설명: sTime * 10  OutMin=0  OutMax=0.000714286
      settings: AttributesFormatString=%<Description>
  sSpdRef : Inport  Description=■ 설명: Speed Reference  Port=2  OutMin=0  OutMax=11000
      settings: AttributesFormatString=%<Description>
  mSMDE_sSpdRefInSeqOut : Inport  Description=■ 설명: Speed Reference Slop Out  Port=3  OutMin=0  OutMax=11000
      settings: AttributesFormatString=%<Description>
  mMCVG_sSpdSlopRising : Inport  Description=■ 설명: Speed Slop Rising Gain  Port=4  OutMin=0  OutMax=3000
      settings: AttributesFormatString=%<Description>
  mMCVG_sSpdSlopFalling : Inport  Description=■ 설명: Speed Slop Falling Gain  Port=5  OutMin=0  OutMax=3000
      settings: AttributesFormatString=%<Description>
  mSMDE_sSpdLimit : Inport  Description=■ 설명: 속도 제한값  Port=6
      settings: AttributesFormatString=%<Description>
  ActionPort : ActionPort  ActionPortLabel=elseif(u2 == 1)
  Nftn_GensAppIeSpdRefLim : Subsystem
  Nftn_SftMdeSpdStart : Subsystem
      settings: RTWFcnNameOpts=Use subsystem name
  mCTRL_sSpdRefIn : Outport  Description=■ 설명: Speed Reference  OutMin=0  OutMax=11000
      settings: AttributesFormatString=%<Description>
  wires:
  Nftn_SftMdeSpdStart/1(mCTRL_sSpdRefIn) -> mCTRL_sSpdRefIn/1
  Nftn_GensAppIeSpdRefLim/1(sSpdRefLimited) -> Nftn_SftMdeSpdStart/1(sSpdRefLimited)
  mBSW_sOutloopTime/1 -> Nftn_SftMdeSpdStart/5(mBSW_sOutloopTime)
  sSpdRef/1 -> Nftn_GensAppIeSpdRefLim/2(sSpdRef)
  mSMDE_sSpdRefInSeqOut/1 -> Nftn_SftMdeSpdStart/2(mSMDE_sSpdRefInSeqOut)
  mMCVG_sSpdSlopRising/1 -> Nftn_SftMdeSpdStart/3(mMCVG_sSpdSlopRising)
  mMCVG_sSpdSlopFalling/1 -> Nftn_SftMdeSpdStart/4(mMCVG_sSpdSlopFalling)
  mSMDE_sSpdLimit/1 -> Nftn_GensAppIeSpdRefLim/1(mSMDE_sSpdLimit)

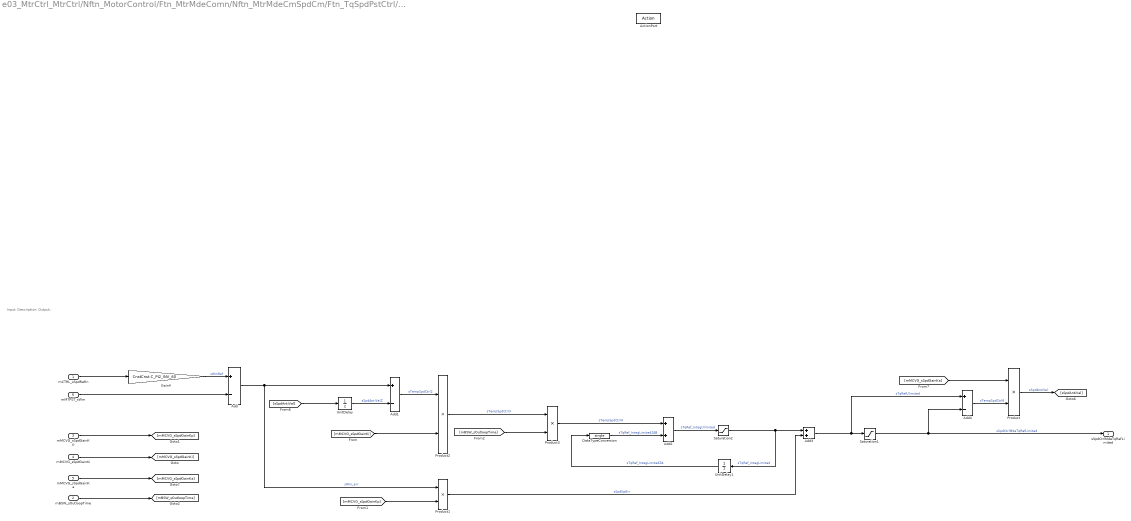
== system e03_MtrCtrl_MtrCtrl/Nftn_MotorControl/Ftn_MtrMdeComn/Nftn_MtrMdeCmSpdCm/Ftn_TqSpdPstCtrl/Ftn_MtrMdeCmSpSpdCtrl/Ftn_SpdCtrl ==
  note: Input:
      | Description:
      | Output:
  mCTRL_sSpdRefIn : Inport  Description=■ 설명: Speed Reference  OutMin=0  OutMax=11000
      settings: AttributesFormatString=%<Description>
  mBSW_sOutloopTime : Inport  Description=■ 설명: sTime * 10  Port=2  OutMin=0  OutMax=0.000714286
      settings: AttributesFormatString=%<Description>
  mMCVG_sSpdGainKp : Inport  Description=■ 설명: Speed Gain Kp Gain  Port=3  OutMin=0  OutMax=10
      settings: AttributesFormatString=%<Description>
  mMCVG_sSpdGainKi : Inport  Description=■ 설명: Speed Gain Ki Gain  Port=4  OutMin=0  OutMax=10
      settings: AttributesFormatString=%<Description>
  mMCVG_sSpdGainKa : Inport  Description=■ 설명: Speed Gain Ka Gain  Port=5  OutMin=0  OutMax=100
      settings: AttributesFormatString=%<Description>
  mMTPST_sWm : Inport  Description=■ 설명: 기계 각속도 (Wm = 12000 * 2pi/60)  Port=6  OutMin=0  OutMax=1256.63706
      settings: AttributesFormatString=%<Description>
  ActionPort : ActionPort  ActionPortLabel=if(u1 == 1)
  Add : Sum  Inputs=+-
  Add1 : Sum  Inputs=+-
  Add2 : Sum
  Add3 : Sum
  Add4 : Sum  Inputs=+-
  DataTypeConversion : DataTypeConversion  OutDataTypeStr=single  SaturateOnIntegerOverflow=off  RndMeth=Floor
  Gain4 : Gain  Gain=CnstCnst.C_PI2_INV_60
  Product{,1..3} (4 alike) : Product
  Saturation1 : Saturate  UpperLimit=E03LIM.sMaxTqSet  LowerLimit=E03LIM.sNegMaxTqSet
      settings: AttributesFormatString=|
      | %<LowerLimit>
      | %<UpperLimit>
  Saturation2 : Saturate  UpperLimit=E03LIM.sMaxTqSet  LowerLimit=E03LIM.sNegMaxTqSet
      settings: AttributesFormatString=|
      | %<LowerLimit>
      | %<UpperLimit>
  UnitDelay : UnitDelay  SampleTime=-1  StateName=sSpdAntiValZ  HasFrameUpgradeWarning=on
  UnitDelay1 : UnitDelay  InitialCondition=E03INIT.sTqRefInit  SampleTime=-1  StateName=sTqRef_IntegZ  HasFrameUpgradeWarning=on
      settings: AttributesFormatString=%<InitialCondition>
  sSpdCtrlMdeTqRefLimited : Outport  Description=■ 설명: 속도 제어기 PI제어 출력값  OutMin=-12577.8  OutMax=12577.8  VectorParamsAs1DForOutWhenUnconnected=off
      settings: AttributesFormatString=%<Description>
  wires:
  Saturation2/1 -> UnitDelay1/1, Add3/1  "sTqRef_IntegLimited"
  Add/1 -> Product1/1, Add1/1  "sWm_err"
  mCTRL_sSpdRefIn/1 -> Gain4/1
  Product1/1 -> Add3/2  "sSpdKpErr"
  Product3/1 -> Add2/1  "sTempSpdCtrl4"
  UnitDelay1/1 -> DataTypeConversion/1  "sTqRef_IntegLimitedZA"
  [sSpdAntiVal] -> UnitDelay/1
  [mBSW_sOutloopTime] -> Product3/2
  Gain4/1 -> Add/1  "sWmRef"
  [mMCVG_sSpdGainKp] -> Product1/2
  Product2/1 -> Product3/1  "sTempSpdCtrl3"
  [mMCVG_sSpdGainKi] -> Product2/2
  Add1/1 -> Product2/1  "sTempSpdCtrl2"
  [mMCVG_sSpdGainKa] -> Product/1
  Product/1 -> [sSpdAntiVal]  "sSpdAntiVal"
  Add2/1 -> Saturation2/1  "sTqRef_IntegUlimited"
  Add3/1 -> Add4/1, Saturation1/1  "sTqRefUlimited"
  Add4/1 -> Product/2  "sTempSpdCtrl6"
  UnitDelay/1 -> Add1/2  "sSpdAntiValZ"
  DataTypeConversion/1 -> Add2/2  "sTqRef_IntegLimitedZAB"
  mBSW_sOutloopTime/1 -> [mBSW_sOutloopTime]
  mMCVG_sSpdGainKp/1 -> [mMCVG_sSpdGainKp]
  mMCVG_sSpdGainKi/1 -> [mMCVG_sSpdGainKi]
  mMCVG_sSpdGainKa/1 -> [mMCVG_sSpdGainKa]
  mMTPST_sWm/1 -> Add/2
  Saturation1/1 -> sSpdCtrlMdeTqRefLimited/1, Add4/2  "sSpdCtrlMdeTqRefLimited"

== system e03_MtrCtrl_MtrCtrl/Nftn_MotorControl/Ftn_MtrMdeComn/Nftn_MtrMdeCmSpdCm/Ftn_TqSpdPstCtrl/Ftn_MtrMdeCmSpSpdCtrl/Subsystem ==
  note: Input:
      | Description:
      | Output:
  ActionPort : ActionPort  ActionPortLabel=else

== system e03_MtrCtrl_MtrCtrl/Nftn_MotorControl/Ftn_MtrMdeComn/Nftn_MtrMdeCmSpdCm/Ftn_TqSpdPstCtrl/Nftn_MtrMdeCmSpdCmTqCtrl/Nftn_SftMdeTqRef ==
  note: Input:
      | Description:
      | Output:
  TqRefLimited : Inport
  mBSW_sTime : Inport  Port=2
  mMCVG_sTqSlpRising : Inport  Port=3
  mMCVG_sTqSlpFalling : Inport  Port=4
  Product : Product
  Product1 : Product
  RelationalOperator1 : RelationalOperator  Operator=<  InputSameDT=off
  RelationalOperator2 : RelationalOperator  Operator=>  InputSameDT=off
  Sum : Sum
  Sum1 : Sum  Inputs=+-
  Switch1 : Switch  Criteria=u2 ~= 0  SaturateOnIntegerOverflow=off  InputSameDT=off
  Switch2 : Switch  Criteria=u2 ~= 0  SaturateOnIntegerOverflow=off  InputSameDT=off
  UnitDelay_sIsRefIn : UnitDelay  InitialCondition=E03INIT.sIsRefInZ  SampleTime=-1  StateName=sIsRefIn2  HasFrameUpgradeWarning=on
      settings: AttributesFormatString=%<InitialCondition>
  mCTRL_sTqRefIn : Outport  VectorParamsAs1DForOutWhenUnconnected=off
  wires:
  UnitDelay_sIsRefIn/1 -> [sIsRefIn2Z]  "sIsRefIn2Z"
  Switch2/1 -> UnitDelay_sIsRefIn/1, mCTRL_sTqRefIn/1  "mCTRL_sTqRefIn"
  TqRefLimited/1 -> RelationalOperator1/1, Switch1/1
  Switch1/1 -> Switch2/1, RelationalOperator2/1  "sBudMax2"
  [sIsRefIn2Z] -> Sum1/1, Sum/2
  Sum1/1 -> RelationalOperator2/2, Switch2/3  "sBaudMin"
  RelationalOperator1/1 -> Switch1/2  "sTempSftCurr1"
  RelationalOperator2/1 -> Switch2/2  "sTempSftCurr2"
  Product1/1 -> Sum1/2  "sStepFalling"
  Product/1 -> Sum/1  "sStepRising"
  Sum/1 -> RelationalOperator1/2, Switch1/3  "sBaudMax1"
  mMCVG_sTqSlpFalling/1 -> Product1/2
  mMCVG_sTqSlpRising/1 -> Product/2
  [mBSW_sTime] -> Product1/1
  mBSW_sTime/1 -> [mBSW_sTime], Product/1

== system e03_MtrCtrl_MtrCtrl/Nftn_MotorControl/Ftn_MtrMdeComn/Nftn_MtrMdeCmSpdCm/Ftn_TqSpdPstCtrl/Nftn_MtrMdeCmSpdCmTqCtrl/Nftn_TqLimit ==
  mCTRL_sTqRefIn : Inport
  bMCEST : Inport  Port=2
  BusSelector : BusSelector  OutputSignals=mMTPST_sIde,mMTPST_sIqe,mMTPST_sTheta
  Gain : Gain  Gain=E03MCMV.sInvKt
  Mux : Mux
  Saturation : Saturate  UpperLimit=E03LIM.sCurrLim  LowerLimit=E03LIM.sNegCurrLim
      settings: AttributesFormatString=|
      | %<LowerLimit>
      | %<UpperLimit>
  sIsRefIdqeTheta5 : Outport
  wires:
  Gain/1 -> Saturation/1  "sCrtRef"
  bMCEST/1 -> BusSelector/1
  BusSelector/1 -> Mux/2  "<mMTPST_sIde>"
  BusSelector/3 -> Mux/4  "<mMTPST_sTheta>"
  Saturation/1 -> Mux/1
  Mux/1 -> sIsRefIdqeTheta5/1  "sIsRefIdqeTheta5"
  BusSelector/2 -> Mux/3  "<mMTPST_sIqe>"
  mCTRL_sTqRefIn/1 -> Gain/1

== system e03_MtrCtrl_MtrCtrl/Nftn_MotorControl/Ftn_MtrMdeComn/Nftn_MtrMdeCmSpdCm/Ftn_TqSpdPstCtrl/Ftn_MtrMdeCmSpSpdCtrl/Ftn_SoftSpdMde/Nftn_GensAppIeSpdRefLim ==
  note: Input:
      | Description:
      | Output:
  mSMDE_sSpdLimit : Inport
  sSpdRef : Inport  Port=2
  Chart_GensAppIeSpdRefLim : Stateflow chart  TreatAsAtomicUnit=on
  sSpdRefLimited : Outport
  wires:
  mSMDE_sSpdLimit/1 -> Chart_GensAppIeSpdRefLim/2(sSpdLimit)
  sSpdRef/1 -> Chart_GensAppIeSpdRefLim/1(sSpdRef)
  Chart_GensAppIeSpdRefLim/1(sSpdRefLimited) -> sSpdRefLimited/1

== system e03_MtrCtrl_MtrCtrl/Nftn_MotorControl/Ftn_MtrMdeComn/Nftn_MtrMdeCmSpdCm/Ftn_TqSpdPstCtrl/Ftn_MtrMdeCmSpSpdCtrl/Ftn_SoftSpdMde/Nftn_SftMdeSpdStart ==
  note: Input:
      | Description:
      | Output:
  sSpdRefLimited : Inport
  mSMDE_sSpdRefInSeqOut : Inport  Port=2
  mMCVG_sSpdSlopRising : Inport  Port=3
  mMCVG_sSpdSlopFalling : Inport  Port=4
  mBSW_sOutloopTime : Inport  Port=5
  Delay : Delay  DelayLength=1
  Product : Product
  Product1 : Product
  RelationalOperator1 : RelationalOperator  Operator=<  InputSameDT=off
  RelationalOperator2 : RelationalOperator  Operator=>  InputSameDT=off
  Sum : Sum
  Sum1 : Sum  Inputs=+-
  Switch1 : Switch  Criteria=u2 ~= 0  SaturateOnIntegerOverflow=off  InputSameDT=off
  Switch2 : Switch  Criteria=u2 ~= 0  SaturateOnIntegerOverflow=off  InputSameDT=off
  Terminator : Terminator
  mCTRL_sSpdRefIn : Outport  VectorParamsAs1DForOutWhenUnconnected=off
  wires:
  Switch2/1 -> Delay/1, mCTRL_sSpdRefIn/1  "mCTRL_sSpdRefIn"
  sSpdRefLimited/1 -> RelationalOperator1/1, Switch1/1
  Switch1/1 -> Switch2/1, RelationalOperator2/1  "sBudMax2"
  Sum1/1 -> RelationalOperator2/2, Switch2/3  "sBaudMin"
  RelationalOperator1/1 -> Switch1/2  "sTempSftSpd1"
  RelationalOperator2/1 -> Switch2/2  "sTempSftSpd2"
  Product1/1 -> Sum1/2  "sStepFalling"
  Product/1 -> Sum/1  "sStepRising"
  Sum/1 -> RelationalOperator1/2, Switch1/3  "sBaudMax1"
  mMCVG_sSpdSlopFalling/1 -> Product1/2
  mMCVG_sSpdSlopRising/1 -> Product/2
  [mBSW_sOutloopTime] -> Product1/1
  mBSW_sOutloopTime/1 -> Product/1, [mBSW_sOutloopTime]
  [mCTRL_sSpdRefInZ] -> Sum/2, Sum1/1
  mSMDE_sSpdRefInSeqOut/1 -> Terminator/1
  Delay/1 -> [mCTRL_sSpdRefInZ]  "mCTRL_sSpdRefInZ"

== stateflow chart e03_MtrCtrl_MtrCtrl/Nftn_MotorControl/Ftn_MtrMdeComn/Ftn_CurrRefSelection/Nftn_SftCurrMde/Nftn_GensAppIeRefLim/Chart_GensAppIeRefLim ==
  (default) -> (junction 7)
  (junction 7) -> (junction 8) [order 1] : [mCTRL_sIsRef > sCurrLim]
  (junction 7) -> (junction 19) [order 2]
  (junction 8) -> (junction 10) : {
      | sIsRefLimed = sCurrLim;
      | }
  (junction 19) -> (junction 16) [order 1] : [mCTRL_sIsRef < -sCurrLim]
  (junction 19) -> (junction 9) [order 2] : {
      | sIsRefLimed = mCTRL_sIsRef;
      | }
  (junction 16) -> (junction 17) : {
      | sIsRefLimed = -sCurrLim;
      | }
  (junction 17) -> (junction 9)
  (junction 10) -> (junction 17)
  (junction 9) -> (junction 11)
  data: mCTRL_sIsRef input; sCurrLim input; sIsRefLimed output double

== stateflow chart e03_MtrCtrl_MtrCtrl/Nftn_MotorControl/Ftn_MtrMdeComn/Nftn_MtrMdeCmSpdCm/Ftn_TqSpdPstCtrl/Ftn_MtrMdeCmSpSpdCtrl/Ftn_SoftSpdMde/Nftn_GensAppIeSpdRefLim/Chart_GensAppIeSpdRefLim ==
  (default) -> (junction 10)
  (junction 10) -> (junction 11) [order 1] : [sSpdRef > sSpdLimit]
  (junction 10) -> (junction 17) [order 2]
  (junction 11) -> (junction 13) : {
      | sSpdRefLimited = sSpdLimit;
      | }
  (junction 17) -> (junction 19) [order 1] : [sSpdRef < -sSpdLimit]
  (junction 17) -> (junction 12) [order 2] : {
      | sSpdRefLimited = sSpdRef;
      | }
  (junction 19) -> (junction 20) : {
      | sSpdRefLimited = -sSpdLimit;
      | }
  (junction 20) -> (junction 12)
  (junction 13) -> (junction 20)
  (junction 12) -> (junction 14)
  data: sSpdRef input; sSpdLimit input; sSpdRefLimited output double

== stateflow chart e03_MtrCtrl_MtrCtrl/Nftn_MotorControl/Ftn_SelectionCtrlMde/Chart ==
  (default) -> (junction 7)
  (junction 7) -> (junction 8) [order 1] : [mSMDE_uFlagInverterOut == u16True]
  (junction 7) -> (junction 9) [order 2] : {
      | uAppCtrlMde = u16Zero;
      | }
  (junction 8) -> (junction 20)
  (junction 20) -> (junction 22) [order 1] : [mDIAG_uFltStat == u16Zero]
  (junction 20) -> (junction 10) [order 2] : {
      | uAppCtrlMde = u16Zero;
      | }
  (junction 22) -> (junction 23) : {
      | uAppCtrlMde = mSMDE_uMtrCtrlMde;
      | }
  (junction 23) -> (junction 10)
  (junction 10) -> (junction 9)
  (junction 9) -> (junction 11)
  data: mSMDE_uMtrCtrlMde input; mSMDE_uFlagInverterOut input; mDIAG_uFltStat input; uAppCtrlMde output uint16; u16Zero input; u16True input

== stateflow chart e03_MtrCtrl_MtrCtrl/Nftn_MotorControl/Ftn_MtrMdeComn/Ftn_MtrMdeCmIFCtrl/Nftn_MtrMdeCmIFCtrlA/Chart ==
  note: sIfTheta 초기값: 0deg*2*PI()/360 = 4.712389
  (default) -> (junction 16)
  (junction 16) -> (junction 18) [order 1] : [mSMDE_sIfFreqSeqOut < sIfSetFreq]
  (junction 16) -> (junction 20) [order 2] : /* no action */
  (junction 18) -> (junction 19) : {
      | mCTRL_sIfFreq = mSMDE_sIfFreqSeqOut + ((sIfSetFreq*mBSW_sTime)/sIfTsec);
      | }
  (junction 19) -> (junction 20)
  (junction 20) -> (junction 1) : {
      | mCTRL_sIfTheta = sIfThetaZ + (C_PI2 * mCTRL_sIfFreq * mBSW_sTime);
      | }
  (junction 1) -> (junction 5) [order 1] : [mCTRL_sIfTheta > C_PI2]
  (junction 1) -> (junction 2) [order 2] : /* no action */
  (junction 5) -> (junction 13) : {
      | mCTRL_sIfTheta = mCTRL_sIfTheta - C_PI2;
      | }
  (junction 13) -> (junction 2)
  (junction 2) -> (junction 29)
  data: mCTRL_sIfFreq output single; mBSW_sTime input; mSMDE_sIfFreqSeqOut input; sIfSetFreq input; sIfTsec input; C_PI2 input =C_PI2; mCTRL_sIfTheta output single; sIfThetaZ input single

== stateflow chart e03_MtrCtrl_MtrCtrl/Nftn_MotorControl/Ftn_MtrMdeComn/Ftn_CurrRefSelection/Nftn_SftCurrMde/Nftn_CalIsBeta2IdqRef/Chart_CalIsBeta2IdqRef ==
  (default) -> (junction 32)
  (junction 32) -> (junction 198) [order 1] : [uAppCtrlMde == C_MODE256_IF]
  (junction 32) -> (junction 213) [order 2] : {
      | sIFreqBetaCmd = sZero;
      | }
  (junction 198) -> (junction 221) : {
      | temp1 =(sIFreqBetaCmd + C_90) * C_PI2_INV_360;
      | sIFreqBetaCmd = sIFreqBetaCmd + sBetaRiseStep;
      | }
  (junction 213) -> (junction 215) [order 1] : [uAppCtrlMde == C_MODE64_VALIGN]
  (junction 213) -> (junction 15) [order 2] : {
      | temp1 =(mCRX_sFreqBetaCmd + C_90) * C_PI2_INV_360;
      | }
  (junction 215) -> (junction 216) : {
      | temp1 = C_90 * C_PI2_INV_360;
      | }
  (junction 221) -> (junction 223) [order 1] : [sIFreqBetaCmd >= sMaxFreq]
  (junction 221) -> (junction 199) [order 2] : /*No Action*/
  (junction 223) -> (junction 224) : {
      | sIFreqBetaCmd = sMaxFreq;
      | }
  (junction 216) -> (junction 15)
  (junction 199) -> (junction 216)
  (junction 224) -> (junction 199)
  (junction 15) -> (junction 13) : {
      | sIdeRefCurrMde = mCTRL_sIsRefIn * single(cos(temp1));
      | }
  (junction 13) -> (junction 16) : {
      | sIqeRefCurrMde = mCTRL_sIsRefIn * single(sin(temp1));
      | }
  data: mCTRL_sIsRefIn input; sIdeRefCurrMde output single; sIqeRefCurrMde output single; temp1 local single; mCRX_sFreqBetaCmd input; uAppCtrlMde input; C_90 input =C_90; C_MODE64_VALIGN input =C_MODE18_ALIGN; C_MODE256_IF input =C_MODE32_IF; C_PI2_INV_360 input =C_PI2_INV_360; sBetaRiseStep input; sMaxFreq input; sIFreqBetaCmd output single; sZero input

== stateflow chart e03_MtrCtrl_MtrCtrl/Nftn_MotorControl/Ftn_MtrCtrlMdeVFCtrl/Nftn_MuxVFCtrl/Chart_MtrCtrlMdeVFCtrl ==
  (default) -> (junction 34) : {
      | sVfThetaRef = sVfThetaRef + (C_PI2 * mCRX_sFreqBetaCmd * mBSW_sTime);
      | }
  (junction 34) -> (junction 37) [order 1] : [sVfThetaRef > C_PI2]
  (junction 34) -> (junction 28) [order 2] : /* No Action */
  (junction 37) -> (junction 36) : {
      | sVfThetaRef = sVfThetaRef - C_PI2;
      | }
  (junction 36) -> (junction 28)
  (junction 28) -> (junction 15)
  data: mCRX_sFreqBetaCmd input; mBSW_sTime input; sVfThetaRef output single; C_PI2 input =C_PI2
